simulink model "Aearial_Inspection_UAV_Simulation"  (R2023a)
settings: Solver=daessc  StartTime=0.0  StopTime=tf  MaxStep=0.1  MinStep=1e-30  RelTol=1e-4
values from neighbouring files (symbols this model uses):
  arm_start = 0    [InitScript.m]
  X = T*[x0;y0]    [line2circle.m]
undefined symbols (not defined in the file or in its folder): arm_end, DiscIntNeverNeededParam, F, is_gust_active, Light, MIL, Mode, Motor_data, params, Robotic_Arm_ASM_DataFile, Sensor_err, servo_specs, simple_env, stepper, Tm, wind_speed, xStack1, xStack2, Y, Z
libraries: sm_lib x399, nesl_utility x78, simulink x25, dspsrcs4 x16, simulink_extras x8, sharedtransform x7, aerolibwind2 x2, sharedutil x1
(part 11 of 12)

== system Aearial_Inspection_UAV_Simulation/UAV/Robotic Arm/Robotic Arm and Servos/Servo_w3/Subsystem1 ==
  desired_angle : Inport
  Discrete-Time Integrator : DiscreteIntegrator  gainval=1  SampleTime=0.01  ICPrevOutput=DiscIntNeverNeededParam  ICPrevScaledInput=DiscIntNeverNeededParam
  Discrete-Time Integrator1 : DiscreteIntegrator  gainval=1  SampleTime=0.01  ICPrevOutput=DiscIntNeverNeededParam  ICPrevScaledInput=DiscIntNeverNeededParam
  Gain1 : Gain  Gain=w/2
  Gain2 : Gain  Gain=2*w
  Saturation1 : Saturate  UpperLimit=max_vel  LowerLimit=-max_vel  ZeroCross=off
  Saturation2 : Saturate  UpperLimit=max_T/I  LowerLimit=-max_T/I  ZeroCross=off
  Simulink-PS Converter : nesl_utility/Simulink-PS Converter  PhysicalDomain=network_engine_domain  SubClassName=ps_input  LeftPortType=input  RightPortType=output  PseudoPeriodic=off  Frequencies=[]  NoiseDistribution=none  NoiseParameters=[]  Unit=rad  AffineConversion=on  FilteringAndDerivatives=provide  SimscapeFilterOrder=1  InputFilterTimeConstant=0.001  UdotUserProvided=2
  Sum : Sum  Inputs=|+-
  Sum2 : Sum  Inputs=|+-
  torque : PMIOPort  Side=Right
  wires:
  desired_angle/1 -> Sum/1
  Sum/1 -> Gain1/1
  Sum2/1 -> Gain2/1
  Gain1/1 -> Saturation1/1
  Saturation1/1 -> Sum2/1
  Gain2/1 -> Saturation2/1
  Discrete-Time Integrator/1 -> Sum/2, Simulink-PS Converter/1
  Discrete-Time Integrator1/1 -> Simulink-PS Converter/2, Sum2/2, Discrete-Time Integrator/1
  Saturation2/1 -> Simulink-PS Converter/3, Discrete-Time Integrator1/1
  connections:
  Simulink-PS Converter/RConn1 -- torque/RConn1

== system Aearial_Inspection_UAV_Simulation/UAV/Robotic Arm/Robotic Arm and Servos/Subsystem/low_torque_servo_1_RIGID ==
  ReferenceFrame : sm_lib/Frames and Transforms/Reference Frame
  Solid : sm_lib/Body Elements/File Solid  ExtGeomFileName=low_torque_servo_Default_sldprt.STEP  UnitType=FromFile  ExtGeomFileUnits=m  StepReaderType=HEX  ExportConvexHullGeometry=off  InertiaType=Custom  Mass=smiData.Solid(6).mass  MassUnits=kg  CenterOfMass=smiData.Solid(6).CoM  CenterOfMassUnits=mm  MomentsOfInertia=smiData.Solid(6).MoI  MomentsOfInertiaUnits=kg*mm^2  ProductsOfInertia=smiData.Solid(6).PoI  ProductsOfInertiaUnits=kg*mm^2  BasedOnType=DensityFromFile  Density=1000  DensityUnits=kg/m^3  DoExposeReferenceFrame=on  SerializedFrames=<Frames/>  GraphicType=FromGeometry  MarkerShape=Sphere  MarkerSize=10  GraphicVisPropType=SimpleVisualProperties  GraphicDiffuseColor=smiData.Solid(6).color  GraphicSpecularColor=[0.5 0.5 0.5 1.0]  GraphicAmbientColor=[0.15 0.15 0.15 1.0]  GraphicEmissiveColor=[0.0 0.0 0.0 1.0]  GraphicShininess=75  GraphicOpacity=smiData.Solid(6).opacity
  Transform : sm_lib/Frames and Transforms/Rigid Transform  TranslationMethod=Cartesian  TranslationStandardOffset=0  TranslationStandardOffsetUnits=mm  TranslationStandardAxis=+Z  TranslationCartesianOffset=smiData.RigidTransform(24).translation  TranslationCartesianOffsetUnits=mm  TranslationROffset=0  TranslationROffsetUnits=m  TranslationZOffset=0  TranslationZOffsetUnits=m  TranslationThetaOffset=0  TranslationThetaOffsetUnits=deg  RotationMethod=ArbitraryAxis  RotationAngleUnits=rad  RotationStandardAxis=+Z  RotationAngle=smiData.RigidTransform(24).angle  RotationArbitraryAxis=smiData.RigidTransform(24).axis  FollAlignAxisA=+X  BaseAlignAxisA=+Y  FollAlignAxisB=+Y  BaseAlignAxisB=+Z  RotationSequenceAxes=FollowerAxes  RotationSequence=XYX  RotationSequenceAngles=[0 0 0]  RotationSequenceAnglesUnits=deg  RotationMatrix=[1 0 0; 0 1 0; 0 0 1]  Quaternion=[1 0 0 0]
  Transform1 : sm_lib/Frames and Transforms/Rigid Transform  TranslationMethod=Cartesian  TranslationStandardOffset=0  TranslationStandardOffsetUnits=mm  TranslationStandardAxis=+Z  TranslationCartesianOffset=smiData.RigidTransform(25).translation  TranslationCartesianOffsetUnits=mm  TranslationROffset=0  TranslationROffsetUnits=m  TranslationZOffset=0  TranslationZOffsetUnits=m  TranslationThetaOffset=0  TranslationThetaOffsetUnits=deg  RotationMethod=ArbitraryAxis  RotationAngleUnits=rad  RotationStandardAxis=+Z  RotationAngle=smiData.RigidTransform(25).angle  RotationArbitraryAxis=smiData.RigidTransform(25).axis  FollAlignAxisA=+X  BaseAlignAxisA=+Y  FollAlignAxisB=+Y  BaseAlignAxisB=+Z  RotationSequenceAxes=FollowerAxes  RotationSequence=XYX  RotationSequenceAngles=[0 0 0]  RotationSequenceAnglesUnits=deg  RotationMatrix=[1 0 0; 0 1 0; 0 0 1]  Quaternion=[1 0 0 0]
  F1 : PMIOPort  Side=Left
  F : PMIOPort  Port=2  Side=Left
  connections:
  ReferenceFrame/RConn1 -- Solid/RConn1 -- Transform/LConn1 -- Transform1/LConn1
  Transform/RConn1 -- F/RConn1
  Transform1/RConn1 -- F1/RConn1

== system Aearial_Inspection_UAV_Simulation/UAV/Robotic Arm/Robotic Arm and Servos/Subsystem/wrist_2nd_joint_1_RIGID ==
  ReferenceFrame : sm_lib/Frames and Transforms/Reference Frame
  Solid : sm_lib/Body Elements/File Solid  ExtGeomFileName=wrist_2nd_joint_Default_sldprt.STEP  UnitType=FromFile  ExtGeomFileUnits=m  StepReaderType=HEX  ExportConvexHullGeometry=off  InertiaType=Custom  Mass=smiData.Solid(8).mass  MassUnits=kg  CenterOfMass=smiData.Solid(8).CoM  CenterOfMassUnits=mm  MomentsOfInertia=smiData.Solid(8).MoI  MomentsOfInertiaUnits=kg*mm^2  ProductsOfInertia=smiData.Solid(8).PoI  ProductsOfInertiaUnits=kg*mm^2  BasedOnType=DensityFromFile  Density=1000  DensityUnits=kg/m^3  DoExposeReferenceFrame=on  SerializedFrames=<Frames/>  GraphicType=FromGeometry  MarkerShape=Sphere  MarkerSize=10  GraphicVisPropType=SimpleVisualProperties  GraphicDiffuseColor=smiData.Solid(8).color  GraphicSpecularColor=[0.5 0.5 0.5 1.0]  GraphicAmbientColor=[0.15 0.15 0.15 1.0]  GraphicEmissiveColor=[0.0 0.0 0.0 1.0]  GraphicShininess=75  GraphicOpacity=smiData.Solid(8).opacity
  Transform : sm_lib/Frames and Transforms/Rigid Transform  TranslationMethod=Cartesian  TranslationStandardOffset=0  TranslationStandardOffsetUnits=mm  TranslationStandardAxis=+Z  TranslationCartesianOffset=smiData.RigidTransform(26).translation  TranslationCartesianOffsetUnits=mm  TranslationROffset=0  TranslationROffsetUnits=m  TranslationZOffset=0  TranslationZOffsetUnits=m  TranslationThetaOffset=0  TranslationThetaOffsetUnits=deg  RotationMethod=ArbitraryAxis  RotationAngleUnits=rad  RotationStandardAxis=+Z  RotationAngle=smiData.RigidTransform(26).angle  RotationArbitraryAxis=smiData.RigidTransform(26).axis  FollAlignAxisA=+X  BaseAlignAxisA=+Y  FollAlignAxisB=+Y  BaseAlignAxisB=+Z  RotationSequenceAxes=FollowerAxes  RotationSequence=XYX  RotationSequenceAngles=[0 0 0]  RotationSequenceAnglesUnits=deg  RotationMatrix=[1 0 0; 0 1 0; 0 0 1]  Quaternion=[1 0 0 0]
  Transform1 : sm_lib/Frames and Transforms/Rigid Transform  TranslationMethod=Cartesian  TranslationStandardOffset=0  TranslationStandardOffsetUnits=mm  TranslationStandardAxis=+Z  TranslationCartesianOffset=smiData.RigidTransform(27).translation  TranslationCartesianOffsetUnits=mm  TranslationROffset=0  TranslationROffsetUnits=m  TranslationZOffset=0  TranslationZOffsetUnits=m  TranslationThetaOffset=0  TranslationThetaOffsetUnits=deg  RotationMethod=ArbitraryAxis  RotationAngleUnits=rad  RotationStandardAxis=+Z  RotationAngle=smiData.RigidTransform(27).angle  RotationArbitraryAxis=smiData.RigidTransform(27).axis  FollAlignAxisA=+X  BaseAlignAxisA=+Y  FollAlignAxisB=+Y  BaseAlignAxisB=+Z  RotationSequenceAxes=FollowerAxes  RotationSequence=XYX  RotationSequenceAngles=[0 0 0]  RotationSequenceAnglesUnits=deg  RotationMatrix=[1 0 0; 0 1 0; 0 0 1]  Quaternion=[1 0 0 0]
  F : PMIOPort  Side=Left
  F1 : PMIOPort  Port=2  Side=Right
  connections:
  ReferenceFrame/RConn1 -- Solid/RConn1 -- Transform/LConn1 -- Transform1/LConn1
  Transform/RConn1 -- F/RConn1
  Transform1/RConn1 -- F1/RConn1

== system Aearial_Inspection_UAV_Simulation/UAV/Robotic Arm/Robotic Arm and Servos/Subsystem1/Probe_1_RIGID ==
  Cylindrical Solid : sm_lib/Body Elements/Cylindrical Solid  GraphicAmbientColor=[0.15 0.15 0.15 1.0]  BasedOnType=Density  CenterOfMass=[0 0 0]  CenterOfMassUnits=m  GraphicDiffuseColor=[0.5 0.5 0.5]  CylinderLength=0.7  CylinderLengthUnits=m  CylinderRadius=0.004  CylinderRadiusUnits=m  Density=0  DensityUnits=kg/m^3  DoExposeReferenceFrame=on  GraphicEmissiveColor=[0.0 0.0 0.0 1.0]  ExportEntireGeometry=on  SerializedFrames=<Frames/>  MarkerShape=Sphere  MarkerSize=10  GraphicType=FromGeometry  InertiaType=CalculateFromGeometry  Mass=1  MassUnits=kg  MomentsOfInertia=[1 1 1]  MomentsOfInertiaUnits=kg*m^2  GraphicOpacity=1.0  ProductsOfInertia=[0 0 0]  ProductsOfInertiaUnits=kg*m^2  GraphicShininess=75  GraphicSpecularColor=[0.5 0.5 0.5 1.0]  GraphicVisPropType=SimpleVisualProperties
  Mux : Mux  Inputs=3
  Mux1 : Mux
  PS-Simulink Converter{,1..5} (6 alike) : nesl_utility/PS-Simulink Converter  PhysicalDomain=network_engine_domain  SubClassName=ps_output  LeftPortType=input  RightPortType=output  PseudoPeriodic=off  Frequencies=[]  VectorFormat=1-D array  Unit=m  AffineConversion=off
  PS-Simulink Converter6 : nesl_utility/PS-Simulink Converter  PhysicalDomain=network_engine_domain  SubClassName=ps_output  LeftPortType=input  RightPortType=output  PseudoPeriodic=off  Frequencies=[]  VectorFormat=1-D array  Unit=inherit  AffineConversion=off
  ReferenceFrame : sm_lib/Frames and Transforms/Reference Frame
  Rigid Transform : sm_lib/Frames and Transforms/Rigid Transform  Commented=on  TranslationMethod=Cartesian  TranslationStandardOffset=0  TranslationStandardOffsetUnits=m  TranslationStandardAxis=+Z  TranslationCartesianOffset=[-0.705 0 0.02]  TranslationCartesianOffsetUnits=m  TranslationROffset=0  TranslationROffsetUnits=m  TranslationZOffset=0  TranslationZOffsetUnits=m  TranslationThetaOffset=0  TranslationThetaOffsetUnits=deg  RotationMethod=None  RotationAngleUnits=deg  RotationStandardAxis=+Z  RotationAngle=0.0  RotationArbitraryAxis=[0 0 1]  FollAlignAxisA=+X  BaseAlignAxisA=+Y  FollAlignAxisB=+Y  BaseAlignAxisB=+Z  RotationSequenceAxes=FollowerAxes  RotationSequence=XYX  RotationSequenceAngles=[0 0 0]  RotationSequenceAnglesUnits=deg  RotationMatrix=[1 0 0; 0 1 0; 0 0 1]  Quaternion=[1 0 0 0]
  Rigid Transform1 : sm_lib/Frames and Transforms/Rigid Transform  TranslationMethod=Cartesian  TranslationStandardOffset=0  TranslationStandardOffsetUnits=m  TranslationStandardAxis=+Z  TranslationCartesianOffset=[0.0465 0 0.02]  TranslationCartesianOffsetUnits=m  TranslationROffset=0  TranslationROffsetUnits=m  TranslationZOffset=0  TranslationZOffsetUnits=m  TranslationThetaOffset=0  TranslationThetaOffsetUnits=deg  RotationMethod=None  RotationAngleUnits=deg  RotationStandardAxis=+Z  RotationAngle=0.0  RotationArbitraryAxis=[0 0 1]  FollAlignAxisA=+X  BaseAlignAxisA=+Y  FollAlignAxisB=+Y  BaseAlignAxisB=+Z  RotationSequenceAxes=FollowerAxes  RotationSequence=XYX  RotationSequenceAngles=[0 0 0]  RotationSequenceAnglesUnits=deg  RotationMatrix=[1 0 0; 0 1 0; 0 0 1]  Quaternion=[1 0 0 0]
  Rigid Transform2 : sm_lib/Frames and Transforms/Rigid Transform  TranslationMethod=Cartesian  TranslationStandardOffset=0  TranslationStandardOffsetUnits=m  TranslationStandardAxis=+Z  TranslationCartesianOffset=[.3555 0 -0.0195]  TranslationCartesianOffsetUnits=m  TranslationROffset=0  TranslationROffsetUnits=m  TranslationZOffset=0  TranslationZOffsetUnits=m  TranslationThetaOffset=0  TranslationThetaOffsetUnits=deg  RotationMethod=StandardAxis  RotationAngleUnits=deg  RotationStandardAxis=+Y  RotationAngle=90  RotationArbitraryAxis=[0 0 1]  FollAlignAxisA=+X  BaseAlignAxisA=+Y  FollAlignAxisB=+Y  BaseAlignAxisB=+Z  RotationSequenceAxes=FollowerAxes  RotationSequence=XYX  RotationSequenceAngles=[0 0 0]  RotationSequenceAnglesUnits=deg  RotationMatrix=[1 0 0; 0 1 0; 0 0 1]  Quaternion=[1 0 0 0]
  Solid : sm_lib/Body Elements/File Solid  ExtGeomFileName=Probe_Default_sldprt.STEP  UnitType=FromFile  ExtGeomFileUnits=m  StepReaderType=HEX  ExportConvexHullGeometry=off  InertiaType=Custom  Mass=smiData.Solid(3).mass  MassUnits=kg  CenterOfMass=smiData.Solid(3).CoM  CenterOfMassUnits=mm  MomentsOfInertia=smiData.Solid(3).MoI  MomentsOfInertiaUnits=kg*mm^2  ProductsOfInertia=smiData.Solid(3).PoI  ProductsOfInertiaUnits=kg*mm^2  BasedOnType=DensityFromFile  Density=1000  DensityUnits=kg/m^3  DoExposeReferenceFrame=on  SerializedFrames=<Frames/>  GraphicType=FromGeometry  MarkerShape=Sphere  MarkerSize=10  GraphicVisPropType=SimpleVisualProperties  GraphicDiffuseColor=smiData.Solid(3).color  GraphicSpecularColor=[0.5 0.5 0.5 1.0]  GraphicAmbientColor=[0.15 0.15 0.15 1.0]  GraphicEmissiveColor=[0.0 0.0 0.0 1.0]  GraphicShininess=75  GraphicOpacity=smiData.Solid(3).opacity
  Transform : sm_lib/Frames and Transforms/Rigid Transform  TranslationMethod=Cartesian  TranslationStandardOffset=0  TranslationStandardOffsetUnits=mm  TranslationStandardAxis=+Z  TranslationCartesianOffset=smiData.RigidTransform(17).translation  TranslationCartesianOffsetUnits=mm  TranslationROffset=0  TranslationROffsetUnits=m  TranslationZOffset=0  TranslationZOffsetUnits=m  TranslationThetaOffset=0  TranslationThetaOffsetUnits=deg  RotationMethod=ArbitraryAxis  RotationAngleUnits=rad  RotationStandardAxis=+Z  RotationAngle=smiData.RigidTransform(17).angle  RotationArbitraryAxis=smiData.RigidTransform(17).axis  FollAlignAxisA=+X  BaseAlignAxisA=+Y  FollAlignAxisB=+Y  BaseAlignAxisB=+Z  RotationSequenceAxes=FollowerAxes  RotationSequence=XYX  RotationSequenceAngles=[0 0 0]  RotationSequenceAnglesUnits=deg  RotationMatrix=[1 0 0; 0 1 0; 0 0 1]  Quaternion=[1 0 0 0]
  Transform Sensor : sm_lib/Frames and Transforms/Transform Sensor  Commented=on  MeasurementFrame=World  RotationSequence=XYX  SenseAngle=off  SenseAxis=off  SenseQ=off  SenseR=off  SenseRotationSequence=off  SenseOmegaX=off  SenseOmegaY=off  SenseOmegaZ=off  SenseQDot=off  SenseRDot=off  SenseRotationSequenceDot=off  SenseAlphaX=off  SenseAlphaY=off  SenseAlphaZ=off  SenseQDDot=off  SenseRDDot=off  SenseX=on  SenseY=on  SenseZ=on  SenseRad=off  SenseAzim=off  SenseDist=off  SenseInc=off  SenseXDot=off  SenseYDot=off  SenseZDot=off  SenseRadDot=off  SenseAzimDot=off  SenseDistDot=off  SenseIncDot=off  SenseXDDot=off  SenseYDDot=off  SenseZDDot=off  SenseRadDDot=off  SenseAzimDDot=off  SenseDistDDot=off  SenseIncDDot=off
  Transform Sensor1 : sm_lib/Frames and Transforms/Transform Sensor  MeasurementFrame=World  RotationSequence=XYX  SenseAngle=off  SenseAxis=off  SenseQ=on  SenseR=off  SenseRotationSequence=off  SenseOmegaX=off  SenseOmegaY=off  SenseOmegaZ=off  SenseQDot=off  SenseRDot=off  SenseRotationSequenceDot=off  SenseAlphaX=off  SenseAlphaY=off  SenseAlphaZ=off  SenseQDDot=off  SenseRDDot=off  SenseX=on  SenseY=on  SenseZ=on  SenseRad=off  SenseAzim=off  SenseDist=off  SenseInc=off  SenseXDot=off  SenseYDot=off  SenseZDot=off  SenseRadDot=off  SenseAzimDot=off  SenseDistDot=off  SenseIncDot=off  SenseXDDot=off  SenseYDDot=off  SenseZDDot=off  SenseRadDDot=off  SenseAzimDDot=off  SenseDistDDot=off  SenseIncDDot=off
  F : PMIOPort  Side=Left
  Prob Geo : PMIOPort  Port=2  Side=Left
  prob head : PMIOPort  Port=3  Side=Left
  prob_disk : PMIOPort  Port=4  Side=Left
  probHeadPos (disconnected) : Outport
  probDiskPos : Outport  Port=2
  wires:
  PS-Simulink Converter/1 -> Mux/1
  PS-Simulink Converter1/1 -> Mux/2
  PS-Simulink Converter2/1 -> Mux/3
  Mux/1 -> probHeadPos (disconnected)/1
  Mux1/1 -> probDiskPos/1
  PS-Simulink Converter5/1 -> Mux1/4
  PS-Simulink Converter4/1 -> Mux1/3
  PS-Simulink Converter3/1 -> Mux1/2
  PS-Simulink Converter6/1 -> Mux1/1
  connections:
  ReferenceFrame/RConn1 -- Rigid Transform1/RConn1 -- Rigid Transform/RConn1 -- Solid/RConn1 -- Rigid Transform2/LConn1 -- Transform/LConn1
  Transform/RConn1 -- F/RConn1
  prob head/RConn1 -- Transform Sensor1/LConn1 -- Transform Sensor/LConn1
  Rigid Transform/LConn1 -- Transform Sensor/RConn1
  PS-Simulink Converter/LConn1 -- Transform Sensor/RConn2
  PS-Simulink Converter1/LConn1 -- Transform Sensor/RConn3
  PS-Simulink Converter2/LConn1 -- Transform Sensor/RConn4
  Transform Sensor1/RConn4 -- PS-Simulink Converter4/LConn1
  Transform Sensor1/RConn3 -- PS-Simulink Converter3/LConn1
  Transform Sensor1/RConn5 -- PS-Simulink Converter5/LConn1
  Transform Sensor1/RConn1 -- prob_disk/RConn1 -- Rigid Transform1/LConn1
  PS-Simulink Converter6/LConn1 -- Transform Sensor1/RConn2
  Cylindrical Solid/RConn1 -- Rigid Transform2/RConn1
  Prob Geo/RConn1 -- Cylindrical Solid/LConn1

== system Aearial_Inspection_UAV_Simulation/UAV/Robotic Arm/Robotic Arm and Servos/Subsystem1/wrist_Cross_Servo_Gear_1_RIGID ==
  ReferenceFrame : sm_lib/Frames and Transforms/Reference Frame
  Solid : sm_lib/Body Elements/File Solid  ExtGeomFileName=wrist_Cross_Servo_Gear_Default_sldprt.STEP  UnitType=FromFile  ExtGeomFileUnits=m  StepReaderType=HEX  ExportConvexHullGeometry=off  InertiaType=Custom  Mass=smiData.Solid(4).mass  MassUnits=kg  CenterOfMass=smiData.Solid(4).CoM  CenterOfMassUnits=mm  MomentsOfInertia=smiData.Solid(4).MoI  MomentsOfInertiaUnits=kg*mm^2  ProductsOfInertia=smiData.Solid(4).PoI  ProductsOfInertiaUnits=kg*mm^2  BasedOnType=DensityFromFile  Density=1000  DensityUnits=kg/m^3  DoExposeReferenceFrame=on  SerializedFrames=<Frames/>  GraphicType=FromGeometry  MarkerShape=Sphere  MarkerSize=10  GraphicVisPropType=SimpleVisualProperties  GraphicDiffuseColor=smiData.Solid(4).color  GraphicSpecularColor=[0.5 0.5 0.5 1.0]  GraphicAmbientColor=[0.15 0.15 0.15 1.0]  GraphicEmissiveColor=[0.0 0.0 0.0 1.0]  GraphicShininess=75  GraphicOpacity=smiData.Solid(4).opacity
  Transform : sm_lib/Frames and Transforms/Rigid Transform  TranslationMethod=Cartesian  TranslationStandardOffset=0  TranslationStandardOffsetUnits=mm  TranslationStandardAxis=+Z  TranslationCartesianOffset=smiData.RigidTransform(20).translation  TranslationCartesianOffsetUnits=mm  TranslationROffset=0  TranslationROffsetUnits=m  TranslationZOffset=0  TranslationZOffsetUnits=m  TranslationThetaOffset=0  TranslationThetaOffsetUnits=deg  RotationMethod=ArbitraryAxis  RotationAngleUnits=rad  RotationStandardAxis=+Z  RotationAngle=smiData.RigidTransform(20).angle  RotationArbitraryAxis=smiData.RigidTransform(20).axis  FollAlignAxisA=+X  BaseAlignAxisA=+Y  FollAlignAxisB=+Y  BaseAlignAxisB=+Z  RotationSequenceAxes=FollowerAxes  RotationSequence=XYX  RotationSequenceAngles=[0 0 0]  RotationSequenceAnglesUnits=deg  RotationMatrix=[1 0 0; 0 1 0; 0 0 1]  Quaternion=[1 0 0 0]
  Transform1 : sm_lib/Frames and Transforms/Rigid Transform  TranslationMethod=Cartesian  TranslationStandardOffset=0  TranslationStandardOffsetUnits=mm  TranslationStandardAxis=+Z  TranslationCartesianOffset=smiData.RigidTransform(23).translation  TranslationCartesianOffsetUnits=mm  TranslationROffset=0  TranslationROffsetUnits=m  TranslationZOffset=0  TranslationZOffsetUnits=m  TranslationThetaOffset=0  TranslationThetaOffsetUnits=deg  RotationMethod=ArbitraryAxis  RotationAngleUnits=rad  RotationStandardAxis=+Z  RotationAngle=smiData.RigidTransform(23).angle  RotationArbitraryAxis=smiData.RigidTransform(23).axis  FollAlignAxisA=+X  BaseAlignAxisA=+Y  FollAlignAxisB=+Y  BaseAlignAxisB=+Z  RotationSequenceAxes=FollowerAxes  RotationSequence=XYX  RotationSequenceAngles=[0 0 0]  RotationSequenceAnglesUnits=deg  RotationMatrix=[1 0 0; 0 1 0; 0 0 1]  Quaternion=[1 0 0 0]
  F : PMIOPort  Side=Left
  F1 : PMIOPort  Port=2  Side=Right
  connections:
  ReferenceFrame/RConn1 -- Solid/RConn1 -- Transform/LConn1 -- Transform1/LConn1
  Transform/RConn1 -- F/RConn1
  Transform1/RConn1 -- F1/RConn1

== system Aearial_Inspection_UAV_Simulation/UAV/Robotic Arm/Robotic Arm and Servos/Subsystem1/wrist_head_1_RIGID ==
  ReferenceFrame : sm_lib/Frames and Transforms/Reference Frame
  Rigid Transform : sm_lib/Frames and Transforms/Rigid Transform  TranslationMethod=None  TranslationStandardOffset=0  TranslationStandardOffsetUnits=m  TranslationStandardAxis=+Z  TranslationCartesianOffset=[0 0 0]  TranslationCartesianOffsetUnits=m  TranslationROffset=0  TranslationROffsetUnits=m  TranslationZOffset=0  TranslationZOffsetUnits=m  TranslationThetaOffset=0  TranslationThetaOffsetUnits=deg  RotationMethod=StandardAxis  RotationAngleUnits=deg  RotationStandardAxis=+Z  RotationAngle=180  RotationArbitraryAxis=[0 0 1]  FollAlignAxisA=+X  BaseAlignAxisA=+Y  FollAlignAxisB=+Y  BaseAlignAxisB=+Z  RotationSequenceAxes=FollowerAxes  RotationSequence=XYX  RotationSequenceAngles=[0 0 0]  RotationSequenceAnglesUnits=deg  RotationMatrix=[1 0 0; 0 1 0; 0 0 1]  Quaternion=[1 0 0 0]
  Solid : sm_lib/Body Elements/File Solid  ExtGeomFileName=wrist_head_Default_sldprt.STEP  UnitType=FromFile  ExtGeomFileUnits=m  StepReaderType=HEX  ExportConvexHullGeometry=off  InertiaType=Custom  Mass=smiData.Solid(5).mass  MassUnits=kg  CenterOfMass=smiData.Solid(5).CoM  CenterOfMassUnits=mm  MomentsOfInertia=smiData.Solid(5).MoI  MomentsOfInertiaUnits=kg*mm^2  ProductsOfInertia=smiData.Solid(5).PoI  ProductsOfInertiaUnits=kg*mm^2  BasedOnType=DensityFromFile  Density=1000  DensityUnits=kg/m^3  DoExposeReferenceFrame=on  SerializedFrames=<Frames/>  GraphicType=FromGeometry  MarkerShape=Sphere  MarkerSize=10  GraphicVisPropType=SimpleVisualProperties  GraphicDiffuseColor=smiData.Solid(5).color  GraphicSpecularColor=[0.5 0.5 0.5 1.0]  GraphicAmbientColor=[0.15 0.15 0.15 1.0]  GraphicEmissiveColor=[0.0 0.0 0.0 1.0]  GraphicShininess=75  GraphicOpacity=smiData.Solid(5).opacity
  Transform : sm_lib/Frames and Transforms/Rigid Transform  TranslationMethod=Cartesian  TranslationStandardOffset=0  TranslationStandardOffsetUnits=mm  TranslationStandardAxis=+Z  TranslationCartesianOffset=smiData.RigidTransform(18).translation  TranslationCartesianOffsetUnits=mm  TranslationROffset=0  TranslationROffsetUnits=m  TranslationZOffset=0  TranslationZOffsetUnits=m  TranslationThetaOffset=0  TranslationThetaOffsetUnits=deg  RotationMethod=ArbitraryAxis  RotationAngleUnits=rad  RotationStandardAxis=+Z  RotationAngle=smiData.RigidTransform(18).angle  RotationArbitraryAxis=smiData.RigidTransform(18).axis  FollAlignAxisA=+X  BaseAlignAxisA=+Y  FollAlignAxisB=+Y  BaseAlignAxisB=+Z  RotationSequenceAxes=FollowerAxes  RotationSequence=XYX  RotationSequenceAngles=[0 0 0]  RotationSequenceAnglesUnits=deg  RotationMatrix=[1 0 0; 0 1 0; 0 0 1]  Quaternion=[1 0 0 0]
  Transform1 : sm_lib/Frames and Transforms/Rigid Transform  TranslationMethod=Cartesian  TranslationStandardOffset=0  TranslationStandardOffsetUnits=mm  TranslationStandardAxis=+Z  TranslationCartesianOffset=smiData.RigidTransform(19).translation  TranslationCartesianOffsetUnits=mm  TranslationROffset=0  TranslationROffsetUnits=m  TranslationZOffset=0  TranslationZOffsetUnits=m  TranslationThetaOffset=0  TranslationThetaOffsetUnits=deg  RotationMethod=ArbitraryAxis  RotationAngleUnits=rad  RotationStandardAxis=+Z  RotationAngle=smiData.RigidTransform(19).angle  RotationArbitraryAxis=smiData.RigidTransform(19).axis  FollAlignAxisA=+X  BaseAlignAxisA=+Y  FollAlignAxisB=+Y  BaseAlignAxisB=+Z  RotationSequenceAxes=FollowerAxes  RotationSequence=XYX  RotationSequenceAngles=[0 0 0]  RotationSequenceAnglesUnits=deg  RotationMatrix=[1 0 0; 0 1 0; 0 0 1]  Quaternion=[1 0 0 0]
  Transform2 : sm_lib/Frames and Transforms/Rigid Transform  TranslationMethod=Cartesian  TranslationStandardOffset=0  TranslationStandardOffsetUnits=mm  TranslationStandardAxis=+Z  TranslationCartesianOffset=smiData.RigidTransform(21).translation  TranslationCartesianOffsetUnits=mm  TranslationROffset=0  TranslationROffsetUnits=m  TranslationZOffset=0  TranslationZOffsetUnits=m  TranslationThetaOffset=0  TranslationThetaOffsetUnits=deg  RotationMethod=ArbitraryAxis  RotationAngleUnits=rad  RotationStandardAxis=+Z  RotationAngle=smiData.RigidTransform(21).angle  RotationArbitraryAxis=smiData.RigidTransform(21).axis  FollAlignAxisA=+X  BaseAlignAxisA=+Y  FollAlignAxisB=+Y  BaseAlignAxisB=+Z  RotationSequenceAxes=FollowerAxes  RotationSequence=XYX  RotationSequenceAngles=[0 0 0]  RotationSequenceAnglesUnits=deg  RotationMatrix=[1 0 0; 0 1 0; 0 0 1]  Quaternion=[1 0 0 0]
  F2 : PMIOPort  Side=Left
  F : PMIOPort  Port=2  Side=Left
  F1 : PMIOPort  Port=3  Side=Right
  connections:
  ReferenceFrame/RConn1 -- Transform1/LConn1 -- Transform2/LConn1 -- Transform/LConn1 -- Solid/RConn1
  Transform/RConn1 -- F/RConn1
  Transform2/RConn1 -- F2/RConn1
  Rigid Transform/RConn1 -- Transform1/RConn1
  Rigid Transform/LConn1 -- F1/RConn1

== system Aearial_Inspection_UAV_Simulation/UAV/Robotic Arm/Robotic Arm and Servos/Subsystem1/wrist_head_cap_1_RIGID ==
  ReferenceFrame : sm_lib/Frames and Transforms/Reference Frame
  Solid : sm_lib/Body Elements/File Solid  ExtGeomFileName=wrist_head_cap_Default_sldprt.STEP  UnitType=FromFile  ExtGeomFileUnits=m  StepReaderType=HEX  ExportConvexHullGeometry=off  InertiaType=Custom  Mass=smiData.Solid(2).mass  MassUnits=kg  CenterOfMass=smiData.Solid(2).CoM  CenterOfMassUnits=mm  MomentsOfInertia=smiData.Solid(2).MoI  MomentsOfInertiaUnits=kg*mm^2  ProductsOfInertia=smiData.Solid(2).PoI  ProductsOfInertiaUnits=kg*mm^2  BasedOnType=DensityFromFile  Density=1000  DensityUnits=kg/m^3  DoExposeReferenceFrame=on  SerializedFrames=<Frames/>  GraphicType=FromGeometry  MarkerShape=Sphere  MarkerSize=10  GraphicVisPropType=SimpleVisualProperties  GraphicDiffuseColor=smiData.Solid(2).color  GraphicSpecularColor=[0.5 0.5 0.5 1.0]  GraphicAmbientColor=[0.15 0.15 0.15 1.0]  GraphicEmissiveColor=[0.0 0.0 0.0 1.0]  GraphicShininess=75  GraphicOpacity=smiData.Solid(2).opacity
  Transform : sm_lib/Frames and Transforms/Rigid Transform  TranslationMethod=Cartesian  TranslationStandardOffset=0  TranslationStandardOffsetUnits=mm  TranslationStandardAxis=+Z  TranslationCartesianOffset=smiData.RigidTransform(22).translation  TranslationCartesianOffsetUnits=mm  TranslationROffset=0  TranslationROffsetUnits=m  TranslationZOffset=0  TranslationZOffsetUnits=m  TranslationThetaOffset=0  TranslationThetaOffsetUnits=deg  RotationMethod=ArbitraryAxis  RotationAngleUnits=rad  RotationStandardAxis=+Z  RotationAngle=smiData.RigidTransform(22).angle  RotationArbitraryAxis=smiData.RigidTransform(22).axis  FollAlignAxisA=+X  BaseAlignAxisA=+Y  FollAlignAxisB=+Y  BaseAlignAxisB=+Z  RotationSequenceAxes=FollowerAxes  RotationSequence=XYX  RotationSequenceAngles=[0 0 0]  RotationSequenceAnglesUnits=deg  RotationMatrix=[1 0 0; 0 1 0; 0 0 1]  Quaternion=[1 0 0 0]
  F : PMIOPort  Side=Left
  connections:
  ReferenceFrame/RConn1 -- Solid/RConn1 -- Transform/LConn1
  Transform/RConn1 -- F/RConn1

== system Aearial_Inspection_UAV_Simulation/UAV/Robotic Arm/Robotic Arm and Servos/Subsystem2/low_torque_servo_2_RIGID ==
  ReferenceFrame : sm_lib/Frames and Transforms/Reference Frame
  Solid : sm_lib/Body Elements/File Solid  ExtGeomFileName=low_torque_servo_Default_sldprt.STEP  UnitType=FromFile  ExtGeomFileUnits=m  StepReaderType=HEX  ExportConvexHullGeometry=off  InertiaType=Custom  Mass=smiData.Solid(6).mass  MassUnits=kg  CenterOfMass=smiData.Solid(6).CoM  CenterOfMassUnits=mm  MomentsOfInertia=smiData.Solid(6).MoI  MomentsOfInertiaUnits=kg*mm^2  ProductsOfInertia=smiData.Solid(6).PoI  ProductsOfInertiaUnits=kg*mm^2  BasedOnType=DensityFromFile  Density=1000  DensityUnits=kg/m^3  DoExposeReferenceFrame=on  SerializedFrames=<Frames/>  GraphicType=FromGeometry  MarkerShape=Sphere  MarkerSize=10  GraphicVisPropType=SimpleVisualProperties  GraphicDiffuseColor=smiData.Solid(6).color  GraphicSpecularColor=[0.5 0.5 0.5 1.0]  GraphicAmbientColor=[0.15 0.15 0.15 1.0]  GraphicEmissiveColor=[0.0 0.0 0.0 1.0]  GraphicShininess=75  GraphicOpacity=smiData.Solid(6).opacity
  Transform : sm_lib/Frames and Transforms/Rigid Transform  TranslationMethod=Cartesian  TranslationStandardOffset=0  TranslationStandardOffsetUnits=mm  TranslationStandardAxis=+Z  TranslationCartesianOffset=smiData.RigidTransform(28).translation  TranslationCartesianOffsetUnits=mm  TranslationROffset=0  TranslationROffsetUnits=m  TranslationZOffset=0  TranslationZOffsetUnits=m  TranslationThetaOffset=0  TranslationThetaOffsetUnits=deg  RotationMethod=ArbitraryAxis  RotationAngleUnits=rad  RotationStandardAxis=+Z  RotationAngle=smiData.RigidTransform(28).angle  RotationArbitraryAxis=smiData.RigidTransform(28).axis  FollAlignAxisA=+X  BaseAlignAxisA=+Y  FollAlignAxisB=+Y  BaseAlignAxisB=+Z  RotationSequenceAxes=FollowerAxes  RotationSequence=XYX  RotationSequenceAngles=[0 0 0]  RotationSequenceAnglesUnits=deg  RotationMatrix=[1 0 0; 0 1 0; 0 0 1]  Quaternion=[1 0 0 0]
  Transform1 : sm_lib/Frames and Transforms/Rigid Transform  TranslationMethod=Cartesian  TranslationStandardOffset=0  TranslationStandardOffsetUnits=mm  TranslationStandardAxis=+Z  TranslationCartesianOffset=smiData.RigidTransform(29).translation  TranslationCartesianOffsetUnits=mm  TranslationROffset=0  TranslationROffsetUnits=m  TranslationZOffset=0  TranslationZOffsetUnits=m  TranslationThetaOffset=0  TranslationThetaOffsetUnits=deg  RotationMethod=ArbitraryAxis  RotationAngleUnits=rad  RotationStandardAxis=+Z  RotationAngle=smiData.RigidTransform(29).angle  RotationArbitraryAxis=smiData.RigidTransform(29).axis  FollAlignAxisA=+X  BaseAlignAxisA=+Y  FollAlignAxisB=+Y  BaseAlignAxisB=+Z  RotationSequenceAxes=FollowerAxes  RotationSequence=XYX  RotationSequenceAngles=[0 0 0]  RotationSequenceAnglesUnits=deg  RotationMatrix=[1 0 0; 0 1 0; 0 0 1]  Quaternion=[1 0 0 0]
  F1 : PMIOPort  Side=Left
  F : PMIOPort  Port=2  Side=Left
  connections:
  ReferenceFrame/RConn1 -- Transform/LConn1 -- Transform1/LConn1 -- Solid/RConn1
  Transform/RConn1 -- F/RConn1
  Transform1/RConn1 -- F1/RConn1

== system Aearial_Inspection_UAV_Simulation/UAV/Robotic Arm/Robotic Arm and Servos/Subsystem2/wrist_1st_joint_1_RIGID ==
  ReferenceFrame : sm_lib/Frames and Transforms/Reference Frame
  Solid : sm_lib/Body Elements/File Solid  ExtGeomFileName=wrist_1st_joint_Default_sldprt.STEP  UnitType=FromFile  ExtGeomFileUnits=m  StepReaderType=HEX  ExportConvexHullGeometry=off  InertiaType=Custom  Mass=smiData.Solid(7).mass  MassUnits=kg  CenterOfMass=smiData.Solid(7).CoM  CenterOfMassUnits=mm  MomentsOfInertia=smiData.Solid(7).MoI  MomentsOfInertiaUnits=kg*mm^2  ProductsOfInertia=smiData.Solid(7).PoI  ProductsOfInertiaUnits=kg*mm^2  BasedOnType=DensityFromFile  Density=1000  DensityUnits=kg/m^3  DoExposeReferenceFrame=on  SerializedFrames=<Frames/>  GraphicType=FromGeometry  MarkerShape=Sphere  MarkerSize=10  GraphicVisPropType=SimpleVisualProperties  GraphicDiffuseColor=smiData.Solid(7).color  GraphicSpecularColor=[0.5 0.5 0.5 1.0]  GraphicAmbientColor=[0.15 0.15 0.15 1.0]  GraphicEmissiveColor=[0.0 0.0 0.0 1.0]  GraphicShininess=75  GraphicOpacity=smiData.Solid(7).opacity
  Transform : sm_lib/Frames and Transforms/Rigid Transform  TranslationMethod=Cartesian  TranslationStandardOffset=0  TranslationStandardOffsetUnits=mm  TranslationStandardAxis=+Z  TranslationCartesianOffset=smiData.RigidTransform(30).translation  TranslationCartesianOffsetUnits=mm  TranslationROffset=0  TranslationROffsetUnits=m  TranslationZOffset=0  TranslationZOffsetUnits=m  TranslationThetaOffset=0  TranslationThetaOffsetUnits=deg  RotationMethod=ArbitraryAxis  RotationAngleUnits=rad  RotationStandardAxis=+Z  RotationAngle=smiData.RigidTransform(30).angle  RotationArbitraryAxis=smiData.RigidTransform(30).axis  FollAlignAxisA=+X  BaseAlignAxisA=+Y  FollAlignAxisB=+Y  BaseAlignAxisB=+Z  RotationSequenceAxes=FollowerAxes  RotationSequence=XYX  RotationSequenceAngles=[0 0 0]  RotationSequenceAnglesUnits=deg  RotationMatrix=[1 0 0; 0 1 0; 0 0 1]  Quaternion=[1 0 0 0]
  Transform1 : sm_lib/Frames and Transforms/Rigid Transform  TranslationMethod=Cartesian  TranslationStandardOffset=0  TranslationStandardOffsetUnits=mm  TranslationStandardAxis=+Z  TranslationCartesianOffset=smiData.RigidTransform(31).translation  TranslationCartesianOffsetUnits=mm  TranslationROffset=0  TranslationROffsetUnits=m  TranslationZOffset=0  TranslationZOffsetUnits=m  TranslationThetaOffset=0  TranslationThetaOffsetUnits=deg  RotationMethod=ArbitraryAxis  RotationAngleUnits=rad  RotationStandardAxis=+Z  RotationAngle=smiData.RigidTransform(31).angle  RotationArbitraryAxis=smiData.RigidTransform(31).axis  FollAlignAxisA=+X  BaseAlignAxisA=+Y  FollAlignAxisB=+Y  BaseAlignAxisB=+Z  RotationSequenceAxes=FollowerAxes  RotationSequence=XYX  RotationSequenceAngles=[0 0 0]  RotationSequenceAnglesUnits=deg  RotationMatrix=[1 0 0; 0 1 0; 0 0 1]  Quaternion=[1 0 0 0]
  F : PMIOPort  Side=Left
  F1 : PMIOPort  Port=2  Side=Right
  connections:
  ReferenceFrame/RConn1 -- Solid/RConn1 -- Transform/LConn1 -- Transform1/LConn1
  Transform/RConn1 -- F/RConn1
  Transform1/RConn1 -- F1/RConn1

== system Aearial_Inspection_UAV_Simulation/UAV/UAV/Body/Drag/Drag Coeficient Selector ==
  u : Inport
  Compare To Constant : simulink/Logic and Bit Operations/Compare To Constant  relop=<=  const=0  OutDataTypeStr=boolean  ZeroCross=off
  Constant : Constant  Value=[-params.CD.front -params.CD.right -params.CD.bottom]
  Constant1 : Constant  Value=[params.CD.back params.CD.left params.CD.top]
  NOT : Logic  Operator=NOT  IconShape=distinctive  AllPortsSameDT=off  OutDataTypeStr=boolean
  Product : Product
  Product3 : Product
  Sum1 : Sum  Inputs=++|
  Out1 : Outport
  wires:
  Compare To Constant/1 -> NOT/1, Product3/2
  Constant/1 -> Product3/1
  Product3/1 -> Sum1/1
  Constant1/1 -> Product/2
  Product/1 -> Sum1/2
  Sum1/1 -> Out1/1
  NOT/1 -> Product/1
  u/1 -> Compare To Constant/1

== system Aearial_Inspection_UAV_Simulation/UAV/UAV/Body/Drag/wind ==
  h : Inport
  UAV Position : Inport  Port=2
  mode : Inport  Port=3
  Constant : Constant  Value=eye(3)
  Constant1 : Constant  Value=5
  Dryden Wind Turbulence Model (Discrete (+q +r)) : aerolibwind2/Dryden Wind Turbulence Model  (Continuous (+q -r))  units=Metric (MKS)  spec=MIL-F-8785C  model=Discrete Dryden (+q +r)  W20=norm(wind_speed)  Wdeg=atan2(wind_speed(2), wind_speed(1))*180/pi+180  TurbProb=10^-2 - Light  L_high=533.4  Wingspan=1  ts=0.3  Seed=[23341 23342 23343 23344]  T_on=on
  Gain : Gain  Gain=is_gust_active
  Gust Manager :) : Subsystem
      settings: PortSchema="{\"entries\":[{\"content\":{\"sides\":[{\"content\":{\"connectorIds\":[\"In1\"]},\"type\":\"ConnectorPlacement.EquallySpacedRectSide\",\"uuid\":\"112b5c87-abfd-4bcb-bbdd-88a8bf3046d7\"},{\"content\":{\"connectorIds\":[],\"side\":\"RIGHT\"},\"type\":\"ConnectorPlacement.EquallySpacedRectSide\",\"uuid\":\"dadb15f0-4966-4df3-b024-5a84aad43b22\"},{\"content\":{\"connectorIds\":[\"Out1\"],\"side\":\"TOP\"},\"type\":\"ConnectorPlacement.EquallySpacedRectSide\",\"uuid\":\"72868ac4-8178-4319-be82-772a1c7bb9d5\"},{\"content\":{\"connectorIds\":[\"In2\",\"In3\"],\"side\":\"BOTTOM\"},\"type\":\"ConnectorPlacement.EquallySpacedRectSide\",\"uuid\":\"1fcf9641-ff38-4f12-9e9f-b839c1abc8f5\"}]},\"type\":\"ConnectorPlacement.EquallySpacedConnector\",\"uuid\":\"34ae4865-4f35-4d2e-b045-e343513b2ddd\"}],\"packageUris\":[\"http://schema.mathworks.com/mf0/Connector/R2020b\"],\"version\":\"1.0\"}"
  Horizontal Wind Model : aerolibwind2/Horizontal Wind Model  units=Metric (MKS)  Vw_source=Internal  Vwind=norm(wind_speed)  W_source=Internal  Wdeg=atan2(wind_speed(2), wind_speed(1))*180/pi+180
  Sum : Sum  Inputs=|++
  Terminator : Terminator
  wind : Outport
  wires:
  Horizontal Wind Model/1 -> Sum/1
  Sum/1 -> wind/1
  Gain/1 -> Sum/2
  Gust Manager :)/1(Out1) -> Gain/1
  h/1 -> Dryden Wind Turbulence Model (Discrete (+q +r))/1
  Constant/1 -> Dryden Wind Turbulence Model (Discrete (+q +r))/3, Horizontal Wind Model/1
  Constant1/1 -> Dryden Wind Turbulence Model (Discrete (+q +r))/2
  Dryden Wind Turbulence Model (Discrete (+q +r))/2 -> Terminator/1
  Dryden Wind Turbulence Model (Discrete (+q +r))/1 -> Gust Manager :)/1(In1)
  UAV Position/1 -> Gust Manager :)/2(UAV Position)
  mode/1 -> Gust Manager :)/3(mode)

== system Aearial_Inspection_UAV_Simulation/UAV/UAV/Body/Drag/wind/Gust Manager :) ==
  In1 : Inport
  UAV Position : Inport  Port=2
  mode : Inport  Port=3
  AND : Logic  IconShape=distinctive  AllPortsSameDT=off  OutDataTypeStr=boolean
  Add Constant : Bias  Bias=[-xStack1 0]  SaturateOnIntegerOverflow=off
  Add Constant1 : Bias  Bias=[-xStack2 0]  SaturateOnIntegerOverflow=off
  Compare To Constant : simulink/Logic and Bit Operations/Compare To Constant  relop===  const=2  OutDataTypeStr=boolean
  Compare To Constant1 : simulink/Logic and Bit Operations/Compare To Constant  relop===  const=5  OutDataTypeStr=boolean
  Compare To Constant2 : simulink/Logic and Bit Operations/Compare To Constant  relop===  const=4  OutDataTypeStr=boolean
  Compare To Constant3 : simulink/Logic and Bit Operations/Compare To Constant  relop===  const=3  OutDataTypeStr=boolean
  Compare To Constant4 : simulink/Logic and Bit Operations/Compare To Constant  relop=<=  const=6  OutDataTypeStr=boolean
  Compare To Constant5 : simulink/Logic and Bit Operations/Compare To Constant  relop=<=  const=6  OutDataTypeStr=boolean
  No Gust : Constant  Value=[0 0 0]
  OR : Logic  Operator=OR  Inputs=4  IconShape=distinctive  AllPortsSameDT=off  OutDataTypeStr=boolean
  OR1 : Logic  Operator=OR  IconShape=distinctive  AllPortsSameDT=off  OutDataTypeStr=boolean
  Selector : Selector  InputPortWidth=3  IndexOptions=Index vector (dialog)  Indices=[1 2]  OutputSizes=1
  Selector1 : Selector  InputPortWidth=3  IndexOptions=Index vector (dialog)  Indices=[1 2]  OutputSizes=1
  Sqrt : Sqrt
  Sqrt1 : Sqrt
  Square : Math  Operator=square
  Square1 : Math  Operator=square
  Sum of Elements : Sum  Inputs=+
  Sum of Elements1 : Sum  Inputs=+
  Switch : Switch  Criteria=u2 > Threshold  SaturateOnIntegerOverflow=off  InputSameDT=off
  Out1 : Outport
  wires:
  No Gust/1 -> Switch/3
  Compare To Constant3/1 -> AND/1
  In1/1 -> Switch/1  "Gust"
  AND/1 -> OR/4
  Compare To Constant/1 -> OR/1
  Compare To Constant2/1 -> OR/3
  Compare To Constant1/1 -> OR/2
  OR/1 -> Switch/2  "gusty condition"
  Switch/1 -> Out1/1
  mode/1 -> Compare To Constant/1, Compare To Constant1/1, Compare To Constant3/1, Compare To Constant2/1
  UAV Position/1 -> Selector1/1, Selector/1
  Selector/1 -> Add Constant/1
  Selector1/1 -> Add Constant1/1
  Add Constant/1 -> Square/1
  Add Constant1/1 -> Square1/1
  Square/1 -> Sum of Elements/1
  Square1/1 -> Sum of Elements1/1
  Sum of Elements/1 -> Sqrt/1
  Sum of Elements1/1 -> Sqrt1/1
  Sqrt/1 -> Compare To Constant4/1
  Sqrt1/1 -> Compare To Constant5/1
  Compare To Constant4/1 -> OR1/1
  Compare To Constant5/1 -> OR1/2
  OR1/1 -> AND/2

== matlab function Aearial_Inspection_UAV_Simulation/Path Palnner/UAV_Guid/Senario 2/senario_2 ==
  data: t input; desired_pos output; desired_psi output; params parameter
function [desired_pos,desired_psi] = senario_2(t, params)

desired_psi = 0;
desired_pos = params.pos0;


end

== matlab function Aearial_Inspection_UAV_Simulation/Path Palnner/UAV_Guid/Senario 1/senario_1 ==
  data: t input; desired_pos output; desired_psi output
function [desired_pos,desired_psi] = senario_1(t)

desired_psi = 0;
desired_pos = [5*sin(t/10) 5*cos(t/10) -t/5];


end

== stateflow chart Aearial_Inspection_UAV_Simulation/Path Palnner/UAV_Guid/Manual/Chart ==
  (default) -> (junction 5)
  (junction 5) -> (junction 7) : [hit]
  (junction 34) -> (junction 123) : {yd = yd - sin(sd);}
  (junction 16) -> (junction 34) : {xd = xd - cos(sd);}
  (junction 7) -> (junction 16) [order 2] : [key == s]
  (junction 7) -> (junction 9) [order 1] : [key == w]
  (junction 9) -> (junction 25) : {xd = xd + cos(sd);}
  (junction 25) -> (junction 115) : {yd = yd + sin(sd);}
  (junction 7) -> (junction 12) [order 3]
  (junction 36) -> (junction 125) : {yd = yd - 5*sin(sd);}
  (junction 18) -> (junction 36) : {xd = xd - 5*cos(sd);}
  (junction 12) -> (junction 18) [order 2] : [key == S]
  (junction 12) -> (junction 14) [order 1] : [key == W]
  (junction 14) -> (junction 28) : {xd = xd + 5*cos(sd);}
  (junction 28) -> (junction 117) : {yd = yd + 5*sin(sd);}
  (junction 12) -> (junction 42) [order 3]
  (junction 50) -> (junction 127) : {xd = xd + sin(sd);}
  (junction 48) -> (junction 50) : {yd = yd - cos(sd);}
  (junction 42) -> (junction 48) [order 2] : [key == a]
  (junction 42) -> (junction 44) [order 1] : [key == d]
  (junction 44) -> (junction 46) : {yd = yd + cos(sd);}
  (junction 46) -> (junction 119) : {xd = xd - sin(sd);}
  (junction 42) -> (junction 54) [order 3]
  (junction 52) -> (junction 129) : {xd = xd + 5*sin(sd);}
  (junction 59) -> (junction 52) : {yd = yd - 5*cos(sd);}
  (junction 54) -> (junction 59) [order 2] : [key == A]
  (junction 54) -> (junction 55) [order 1] : [key == D]
  (junction 55) -> (junction 56) : {yd = yd + 5*cos(sd);}
  (junction 56) -> (junction 121) : {xd = xd - 5*sin(sd);}
  (junction 54) -> (junction 77) [order 3]
  (junction 73) -> (junction 79) : {zd = zd - 1;}
  (junction 77) -> (junction 73) [order 2] : [key == q]
  (junction 77) -> (junction 75) [order 1] : [key == e]
  (junction 75) -> (junction 80) : {zd = zd + 1;}
  (junction 77) -> (junction 64) [order 3]
  (junction 69) -> (junction 62) : {zd = zd - 5;}
  (junction 64) -> (junction 69) [order 2] : [key == Q]
  (junction 64) -> (junction 65) [order 1] : [key == E]
  (junction 65) -> (junction 66) : {zd = zd + 5;}
  (junction 64) -> (junction 95) [order 3]
  (junction 93) -> (junction 99) : {sd = sd - 1*3.14/180;}
  (junction 95) -> (junction 93) [order 2] : [key == z]
  (junction 95) -> (junction 91) [order 1] : [key == x]
  (junction 91) -> (junction 106) : {sd = sd + 1*3.14/180;}
  (junction 95) -> (junction 107) [order 3]
  (junction 103) -> (junction 109) : {sd = sd - 5*3.14/180;}
  (junction 107) -> (junction 103) [order 2] : [key == Z]
  (junction 107) -> (junction 105) [order 1] : [key == X]
  (junction 105) -> (junction 100) : {sd = sd + 5*3.14/180;}
  data: hit input; key input; w constant double =119; a constant double =97; A constant double =65; W constant double =87; s constant double =115; S constant double =83; xd output =0; d constant double =100; e constant double =101; q constant double =113; yd output =0; zd output =0; D constant double =68; E constant double =69; Q constant double =81; sd output =0; x constant double =120; z constant double =122; X constant double =88; Z constant double =90

== matlab function Aearial_Inspection_UAV_Simulation/Path Palnner/UAV_Guid/Senario 3/senario_3 ==
  data: pre_desired_pos input; desired_pos output size=[1 3]; desired_psi output; t input; simple_env parameter; params parameter
function [desired_pos,desired_psi] = senario_3(pre_desired_pos, t, simple_env, params)

wait_time = 3;

if t < wait_time
    desired_pos = params.pos0;
    desired_psi = params.Eul0(3)*pi/180;
else
    t = t - wait_time;
    pos0_x = params.pos0(1);
    pos0_y = params.pos0(2);
    
    xStack1 = simple_env.stack1_x;
    xStack2 = simple_env.stack2_x;
    
    rStack1 = simple_env.stack1_r;
    rStack2 = simple_env.stack2_r;
    
    cOffset = 1.5;
    
    cR1 = rStack1 + cOffset;
    cR2 = rStack2 + cOffset;
    
    [xMerge, yMerge]   =  line2circle(xStack2, 0, cR2, [pos0_x ;pos0_y]);
    [xDetach, yDetach] =  line2circle(xStack2, 0, cR2, [xStack1 + cR1 ;0]);
    
    v = 1;
    aMerge  = yMerge/(xMerge - pos0_x);
    aDetach = yDetach/(-xStack1 - cR1 + xDetach);
    
    x = max(pos0_x-v*t, xStack1 + cR1);
    if(x > xMerge)
        y = aMerge * (x - pos0_x);
        z = 0;
    elseif(x > xDetach)
        y = sqrt(abs(cR2^2 - ((pos0_x-x)-xStack2)^2));
        z = 0;
    else
        y = aDetach * (x - xStack1 - cR1);
        z = 0 + .06*(x-xDetach);
    end
    
    desired_pos = [x, y, z];
    desired_psi = atan2(desired_pos(2) - pre_desired_pos(2), desired_pos(1) - pre_desired_pos(1));
    if abs(desired_psi) < pi/2
        desired_psi = pi;
    end
%     desired_psi = max(0.8*pi,min(1.2*pi, desired_psi));
end
end


function [x,y] = line2circle(x_o,y_o,R, pos)

x0 = x_o - pos(1);
y0 = y_o - pos(2);

theta = abs(atan(y0/x0));
T = [cos(theta) sin(theta);-sin(theta) cos(theta)];

X = T*[x0;y0];
x3 = X(1);

x1  = (x3^2-R^2)/x3;
y1  = sqrt(x3^2-R^2 - x1^2);

x = T(:,1)'*[x1;y1] + pos(1);
y = T(:,2)'*[x1;y1]+pos(2);

end

== matlab function Aearial_Inspection_UAV_Simulation/Path Palnner/UAV_Guid/Senario 4/senario_4 ==
  data: t input; desired_pos output; desired_psi output; simple_env parameter
function [desired_pos,desired_psi] = senario_4(t, simple_env)

rs = simple_env.stack1_r;
cf = simple_env.safty_zone;
zst = 0;
zf  = zst + simple_env.inspection_height;

xe  = -rs-cf;
ye  = 0;
ze  = zf;

t = max(0, t-3);

circle_time = 30;
desired_pos = [(t<circle_time) (t>=circle_time)]*[  (rs + cf)*cos(pi*t/circle_time) -(rs + cf)*sin(pi*t/circle_time)    (ze-zst)*t/circle_time+zst
    xe                                  ye                              ze];
desired_psi = atan2(-desired_pos(2), -desired_pos(1))+2*pi;
end

== matlab function Aearial_Inspection_UAV_Simulation/Path Palnner/UAV_Guid/Senario 5/senario_5 ==
  data: desired_pos output; desired_psi output; t input; params parameter
function [desired_pos,desired_psi] = senario_5(t, params)
start_pos_x = params.pos0(1);
start_pos_z = params.pos0(3);
pos_x_for_inspection = -1.78;

step1_duration = 3;
step2_arrival_des_pos_time = 3;
step2_duration = params.t_flight_toward_flange-step1_duration + params.t_flange_placement + params.t_inspection ...
                + params.t_probe_backward + params.t_probe_down;

% step 1 : stabilization
if t < step1_duration
    desired_psi = 0;
    desired_pos = [start_pos_x 0 start_pos_z];

% step 2 : moving toward flange and stay for inspection
elseif t < step2_duration + step1_duration + 1
    t = t - step1_duration; 
    d_pos_x = pos_x_for_inspection - start_pos_x;
    desired_psi = 0;
    desired_pos = [start_pos_x+d_pos_x*(t < step2_arrival_des_pos_time)*t/step2_arrival_des_pos_time + d_pos_x*(t>=step2_arrival_des_pos_time) 0 start_pos_z];
else
    desired_psi = 0;
    desired_pos = [start_pos_x 0 start_pos_z]; 
end

end

== stateflow chart Aearial_Inspection_UAV_Simulation/Path Palnner/Arm Guid/Manual/Chart ==
  (default) -> (junction 5)
  (junction 5) -> (junction 7) : [hit]
  (junction 34) -> (junction 123) : {yd = yd - sin(sd);}
  (junction 16) -> (junction 34) : {xd = xd - cos(sd);}
  (junction 7) -> (junction 16) [order 2] : [key == s]
  (junction 7) -> (junction 9) [order 1] : [key == w]
  (junction 9) -> (junction 25) : {xd = xd + cos(sd);}
  (junction 25) -> (junction 115) : {yd = yd + sin(sd);}
  (junction 7) -> (junction 12) [order 3]
  (junction 36) -> (junction 125) : {yd = yd - 5*sin(sd);}
  (junction 18) -> (junction 36) : {xd = xd - 5*cos(sd);}
  (junction 12) -> (junction 18) [order 2] : [key == S]
  (junction 12) -> (junction 14) [order 1] : [key == W]
  (junction 14) -> (junction 28) : {xd = xd + 5*cos(sd);}
  (junction 28) -> (junction 117) : {yd = yd + 5*sin(sd);}
  (junction 12) -> (junction 42) [order 3]
  (junction 50) -> (junction 127) : {xd = xd + sin(sd);}
  (junction 48) -> (junction 50) : {yd = yd - cos(sd);}
  (junction 42) -> (junction 48) [order 2] : [key == a]
  (junction 42) -> (junction 44) [order 1] : [key == d]
  (junction 44) -> (junction 46) : {yd = yd + cos(sd);}
  (junction 46) -> (junction 119) : {xd = xd - sin(sd);}
  (junction 42) -> (junction 54) [order 3]
  (junction 52) -> (junction 129) : {xd = xd + 5*sin(sd);}
  (junction 59) -> (junction 52) : {yd = yd - 5*cos(sd);}
  (junction 54) -> (junction 59) [order 2] : [key == A]
  (junction 54) -> (junction 55) [order 1] : [key == D]
  (junction 55) -> (junction 56) : {yd = yd + 5*cos(sd);}
  (junction 56) -> (junction 121) : {xd = xd - 5*sin(sd);}
  (junction 54) -> (junction 77) [order 3]
  (junction 73) -> (junction 79) : {zd = zd - 1;}
  (junction 77) -> (junction 73) [order 2] : [key == q]
  (junction 77) -> (junction 75) [order 1] : [key == e]
  (junction 75) -> (junction 80) : {zd = zd + 1;}
  (junction 77) -> (junction 64) [order 3]
  (junction 69) -> (junction 62) : {zd = zd - 5;}
  (junction 64) -> (junction 69) [order 2] : [key == Q]
  (junction 64) -> (junction 65) [order 1] : [key == E]
  (junction 65) -> (junction 66) : {zd = zd + 5;}
  (junction 64) -> (junction 95) [order 3]
  (junction 93) -> (junction 99) : {sd = sd - 1*3.14/180;}
  (junction 95) -> (junction 93) [order 2] : [key == z]
  (junction 95) -> (junction 91) [order 1] : [key == x]
  (junction 91) -> (junction 106) : {sd = sd + 1*3.14/180;}
  (junction 95) -> (junction 107) [order 3]
  (junction 103) -> (junction 109) : {sd = sd - 5*3.14/180;}
  (junction 107) -> (junction 103) [order 2] : [key == Z]
  (junction 107) -> (junction 105) [order 1] : [key == X]
  (junction 105) -> (junction 100) : {sd = sd + 5*3.14/180;}
  data: hit input; key input; w constant double =119; a constant double =97; A constant double =65; W constant double =87; s constant double =115; S constant double =83; xd output =0; d constant double =100; e constant double =101; q constant double =113; yd output =0; zd output =0; D constant double =68; E constant double =69; Q constant double =81; sd output =0; x constant double =120; z constant double =122; X constant double =88; Z constant double =90

== matlab function Aearial_Inspection_UAV_Simulation/Path Palnner/Arm Guid/Senario 1/senario_1 ==
  data: t input; desired_pos output; desired_psi output
function [desired_pos,desired_psi] = senario_1(t)

desired_psi = 0;
desired_pos = [0 0 0];


end
